simulink model "Exp_3_batch_12_simulation4"  (R2020a)
settings: Solver=VariableStepAuto  StartTime=0.0  StopTime=20  RelTol=1e-3
settings Model: Creator=sundaram bhupathi  LastModifiedBy=sundaram bhupathi

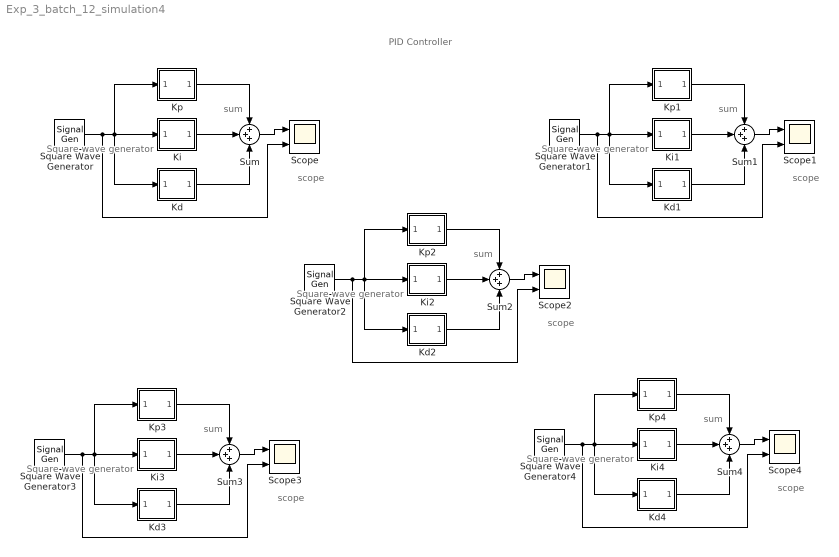
== system Exp_3_batch_12_simulation4 ==
  note: Square wave generator
  note: sum
  note: scope
  note: PID Controller
  note: sum
  note: scope
  note: Square wave generator
  note: sum
  note: scope
  note: Square wave generator
  note: sum
  note: scope
  note: Square wave generator
  note: sum
  note: scope
  note: Square wave generator
  Kd : Subsystem
  Kd1 : Subsystem
  Kd2 : Subsystem
  Kd3 : Subsystem
  Kd4 : Subsystem
  Ki : Subsystem
  Ki1 : Subsystem
  Ki2 : Subsystem
  Ki3 : Subsystem
  Ki4 : Subsystem
  Kp : Subsystem
  Kp1 : Subsystem
  Kp2 : Subsystem
  Kp3 : Subsystem
  Kp4 : Subsystem
  Scope{,1..4} (5 alike) : Scope  NumInputPorts=2
  Square Wave Generator{,1..4} (5 alike) : SignalGenerator  WaveForm=square  Amplitude=10  Units=rad/sec
  Sum{,1..4} (5 alike) : Sum  Inputs=+++  InputSameDT=on  SaturateOnIntegerOverflow=on  OutDataTypeStr=Inherit: Same as first input
  wires:
  Kp/1(Out1) -> Sum/1
  Square Wave Generator/1 -> Scope/2, Kd/1(In1), Ki/1(In1), Kp/1(In1)
  Ki/1(Out1) -> Sum/2
  Sum/1 -> Scope/1
  Kd/1(Out1) -> Sum/3
  Kd1/1(Out1) -> Sum1/3
  Square Wave Generator1/1 -> Scope1/2, Kd1/1(In1), Ki1/1(In1), Kp1/1(In1)
  Kp1/1(Out1) -> Sum1/1
  Ki1/1(Out1) -> Sum1/2
  Sum1/1 -> Scope1/1
  Kd2/1(Out1) -> Sum2/3
  Square Wave Generator2/1 -> Scope2/2, Kd2/1(In1), Ki2/1(In1), Kp2/1(In1)
  Kp2/1(Out1) -> Sum2/1
  Ki2/1(Out1) -> Sum2/2
  Sum2/1 -> Scope2/1
  Kd3/1(Out1) -> Sum3/3
  Square Wave Generator3/1 -> Scope3/2, Kd3/1(In1), Ki3/1(In1), Kp3/1(In1)
  Kp3/1(Out1) -> Sum3/1
  Ki3/1(Out1) -> Sum3/2
  Sum3/1 -> Scope3/1
  Kd4/1(Out1) -> Sum4/3
  Square Wave Generator4/1 -> Scope4/2, Kd4/1(In1), Ki4/1(In1), Kp4/1(In1)
  Kp4/1(Out1) -> Sum4/1
  Ki4/1(Out1) -> Sum4/2
  Sum4/1 -> Scope4/1

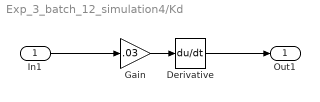
== system Exp_3_batch_12_simulation4/Kd ==
  In1 : Inport
  Derivative : Derivative
  Gain : Gain  Gain=.03
  Out1 : Outport
  wires:
  In1/1 -> Gain/1
  Gain/1 -> Derivative/1
  Derivative/1 -> Out1/1

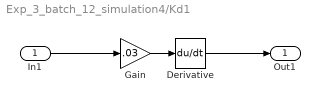
== system Exp_3_batch_12_simulation4/Kd1 ==
  In1 : Inport
  Derivative : Derivative
  Gain : Gain  Gain=.03
  Out1 : Outport
  wires:
  In1/1 -> Gain/1
  Gain/1 -> Derivative/1
  Derivative/1 -> Out1/1

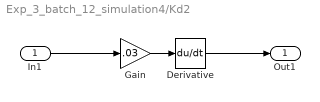
== system Exp_3_batch_12_simulation4/Kd2 ==
  In1 : Inport
  Derivative : Derivative
  Gain : Gain  Gain=.03
  Out1 : Outport
  wires:
  In1/1 -> Gain/1
  Gain/1 -> Derivative/1
  Derivative/1 -> Out1/1

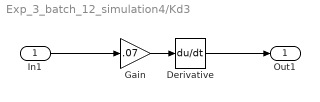
== system Exp_3_batch_12_simulation4/Kd3 ==
  In1 : Inport
  Derivative : Derivative
  Gain : Gain  Gain=.07
  Out1 : Outport
  wires:
  In1/1 -> Gain/1
  Gain/1 -> Derivative/1
  Derivative/1 -> Out1/1

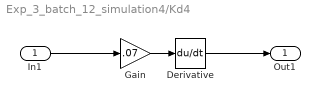
== system Exp_3_batch_12_simulation4/Kd4 ==
  In1 : Inport
  Derivative : Derivative
  Gain : Gain  Gain=.07
  Out1 : Outport
  wires:
  In1/1 -> Gain/1
  Gain/1 -> Derivative/1
  Derivative/1 -> Out1/1

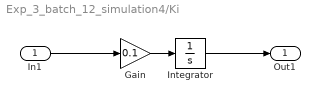
== system Exp_3_batch_12_simulation4/Ki ==
  In1 : Inport
  Gain : Gain  Gain=0.1
  Integrator : Integrator
  Out1 : Outport
  wires:
  In1/1 -> Gain/1
  Gain/1 -> Integrator/1
  Integrator/1 -> Out1/1

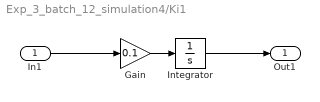
== system Exp_3_batch_12_simulation4/Ki1 ==
  In1 : Inport
  Gain : Gain  Gain=0.1
  Integrator : Integrator
  Out1 : Outport
  wires:
  In1/1 -> Gain/1
  Gain/1 -> Integrator/1
  Integrator/1 -> Out1/1

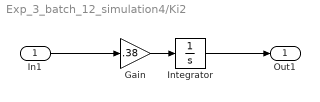
== system Exp_3_batch_12_simulation4/Ki2 ==
  In1 : Inport
  Gain : Gain  Gain=.38
  Integrator : Integrator
  Out1 : Outport
  wires:
  In1/1 -> Gain/1
  Gain/1 -> Integrator/1
  Integrator/1 -> Out1/1

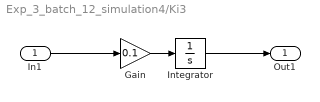
== system Exp_3_batch_12_simulation4/Ki3 ==
  In1 : Inport
  Gain : Gain  Gain=0.1
  Integrator : Integrator
  Out1 : Outport
  wires:
  In1/1 -> Gain/1
  Gain/1 -> Integrator/1
  Integrator/1 -> Out1/1

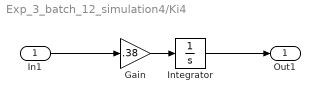
== system Exp_3_batch_12_simulation4/Ki4 ==
  In1 : Inport
  Gain : Gain  Gain=.38
  Integrator : Integrator
  Out1 : Outport
  wires:
  In1/1 -> Gain/1
  Gain/1 -> Integrator/1
  Integrator/1 -> Out1/1

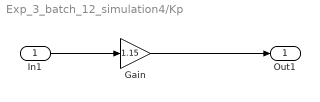
== system Exp_3_batch_12_simulation4/Kp ==
  In1 : Inport
  Gain : Gain  Gain=1.15
  Out1 : Outport
  wires:
  In1/1 -> Gain/1
  Gain/1 -> Out1/1

== system Exp_3_batch_12_simulation4/Kp1 ==
  In1 : Inport
  Gain : Gain  Gain=2
  Out1 : Outport
  wires:
  In1/1 -> Gain/1
  Gain/1 -> Out1/1

== system Exp_3_batch_12_simulation4/Kp2 ==
  In1 : Inport
  Gain : Gain  Gain=1.15
  Out1 : Outport
  wires:
  In1/1 -> Gain/1
  Gain/1 -> Out1/1

== system Exp_3_batch_12_simulation4/Kp3 ==
  In1 : Inport
  Gain : Gain  Gain=1.15
  Out1 : Outport
  wires:
  In1/1 -> Gain/1
  Gain/1 -> Out1/1

== system Exp_3_batch_12_simulation4/Kp4 ==
  In1 : Inport
  Gain : Gain  Gain=2
  Out1 : Outport
  wires:
  In1/1 -> Gain/1
  Gain/1 -> Out1/1
